simulink model "SCwith2SAsaug_ter"  (R2025b)
settings: Solver=VariableStepAuto  StartTime=0.0  StopTime=10.0  RelTol=1e-3
undefined symbols (not defined in the file): InvDyn, sig4, ureal, uss
libraries: RCTblocks x67
(part 1 of 2)
settings Model: Creator=d.alazard  LastModifiedBy=andre
settings SolverCC: AlgebraicLoopSolver=TrustRegion
settings DebuggingCC: AlgebraicLoopMsg=none  UnconnectedInputMsg=warning  UnconnectedOutputMsg=warning  UnconnectedLineMsg=warning
settings ModelReferenceCC: EnableRefExpFcnMdlSchedulingChecks=on
settings RTWCC: GPUComputeCapability=3.5  DLArmComputeVersion=19.05

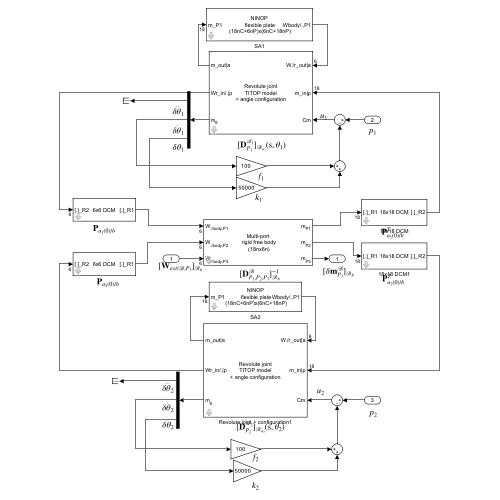
[thumbnail: Simulink's stored preview of the top-level diagram]
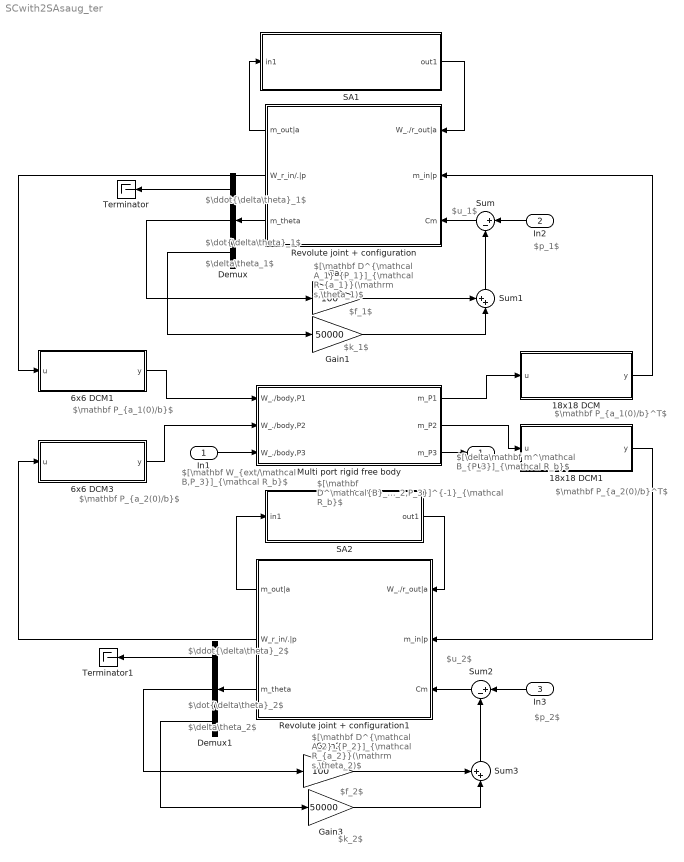
== system SCwith2SAsaug_ter ==
  note: $u_1$
  note: $\ddot{\delta\theta}_1$
  note: $\mathbf P_{a_1(0)/b}^T$
  note: $[\mathbf D^\mathcal{B}_{P_1,P_2,P_3}]^{-1}_{\mathcal R_b}$
  note: $\mathbf P_{a_1(0)/b}$
  note: $\mathbf P_{a_2(0)/b}$
  note: $\mathbf P_{a_2(0)/b}^T$
  note: $\dot{\delta\theta}_1$
  note: $\dot{\delta\theta}_2$
  note: $\ddot{\delta\theta}_2$
  note: $\delta\theta_1$
  note: $\delta\theta_2$
  note: $p_1$
  note: $u_2$
  note: $p_2$
  note: $f_1$
  note: $k_1$
  note: $k_2$
  note: $f_2$
  note: $[\mathbf D^{\mathcal A_1}_{P_1}]_{\mathcal R_{a_1}}(\mathrm s,\theta_1)$
  note: $[\mathbf D^{\mathcal A_2}_{P_2}]_{\mathcal R_{a_2}}(\mathrm s,\theta_2)$
  note: $[\mathbf W_{ext/\mathcal B,P_3}]_{\mathcal R_b}$
  note: $[\delta\mathbf m^\mathcal B_{P_3}]_{\mathcal R_b}$
  In1 : Inport
  In2 : Inport  Port=2
  In3 : Inport  Port=3
  18x18 DCM : Subsystem  mask(18x18 Direction cosine matrix (DCM)){rot=[0 -1 0;0 0 -1;1 0 0], transp=on}
      mask prompts: rot "3x3 DCM"; transp "Matrix transposed"
      mask help:
      | For 6 d.o.f. body motion vector (3 translations and 3 rotations, accelerations, velocities and positions), this block Implement the 18x18 rotation matrix (or its transposed) for a given 3x3 DCM.
      |
      | Considering 2 frames R1 and  R2, the DCM between R1 and R2 is defined as the 3x3 matrix where each column is the component vector of each R2 orthogonal unit vector expressed in R1. Thus
      |
      |    [v]_R1 = DCM  * [v]_R2.
      mask init:
      | if transp,
      |     rot=rot';
      | end
      mask Help: web('Doc18dcm.html','-browser')
      mask Display:
      | disp('18x18 DCM')
      | if transp
      |     port_label('input', 1, '[.]_R1')
      |     port_label('output', 1, '[.]_R2')
      | else
      |     port_label('input', 1, '[.]_R2')
      |     port_label('output', 1, '[.]_R1')
      | end
  18x18 DCM1 : Subsystem  mask(18x18 Direction cosine matrix (DCM)){rot=[0 1 0;0 0 -1;-1 0 0], transp=on}
      mask prompts: rot "3x3 DCM"; transp "Matrix transposed"
      mask help:
      | For 6 d.o.f. body motion vector (3 translations and 3 rotations, accelerations, velocities and positions), this block Implement the 18x18 rotation matrix (or its transposed) for a given 3x3 DCM.
      |
      | Considering 2 frames R1 and  R2, the DCM between R1 and R2 is defined as the 3x3 matrix where each column is the component vector of each R2 orthogonal unit vector expressed in R1. Thus
      |
      |    [v]_R1 = DCM  * [v]_R2.
      mask init:
      | if transp,
      |     rot=rot';
      | end
      mask Help: web('Doc18dcm.html','-browser')
      mask Display:
      | disp('18x18 DCM')
      | if transp
      |     port_label('input', 1, '[.]_R1')
      |     port_label('output', 1, '[.]_R2')
      | else
      |     port_label('input', 1, '[.]_R2')
      |     port_label('output', 1, '[.]_R1')
      | end
  6x6 DCM1 : Subsystem  mask(6x6 Direction cosine matrix (DCM)){rot=[0 -1 0;0 0 -1;1 0 0], transp=off}
      mask prompts: rot "3x3 DCM"; transp "Matrix transposed"
      mask help:
      | For 6 d.o.f. body motion (3 translations and 3 rotations), this block Implement the 6x6 rotation matrix (or its transposed) for a given 3x3 DCM.
      |
      | Considering 2 frames R1 and  R2, the DCM between R1 and R2 is defined as the 3x3 matrix where each column is the component vector of each R2 orthogonal unit vector expressed in R1. Thus
      |
      |    [v]_R1 = DCM  * [v]_R2.
      mask init:
      | if transp,
      |     rot=rot';
      | end
      mask Help: web('Doc6dcm.html','-browser')
      mask Display:
      | disp('6x6 DCM')
      | if transp
      |     port_label('input', 1, '[.]_R1')
      |     port_label('output', 1, '[.]_R2')
      | else
      |     port_label('input', 1, '[.]_R2')
      |     port_label('output', 1, '[.]_R1')
      | end
  6x6 DCM3 : Subsystem  mask(6x6 Direction cosine matrix (DCM)){rot=[0 1 0;0 0 -1;-1 0 0], transp=off}
      mask prompts: rot "3x3 DCM"; transp "Matrix transposed"
      mask help:
      | For 6 d.o.f. body motion (3 translations and 3 rotations), this block Implement the 6x6 rotation matrix (or its transposed) for a given 3x3 DCM.
      |
      | Considering 2 frames R1 and  R2, the DCM between R1 and R2 is defined as the 3x3 matrix where each column is the component vector of each R2 orthogonal unit vector expressed in R1. Thus
      |
      |    [v]_R1 = DCM  * [v]_R2.
      mask init:
      | if transp,
      |     rot=rot';
      | end
      mask Help: web('Doc6dcm.html','-browser')
      mask Display:
      | disp('6x6 DCM')
      | if transp
      |     port_label('input', 1, '[.]_R1')
      |     port_label('output', 1, '[.]_R2')
      | else
      |     port_label('input', 1, '[.]_R2')
      |     port_label('output', 1, '[.]_R1')
      | end
  Demux : Demux  Outputs=3
  Demux1 : Demux  Outputs=3
  Gain : Gain  Gain=100
  Gain1 : Gain  Gain=50000
  Gain2 : Gain  Gain=100
  Gain3 : Gain  Gain=50000
  Multi port rigid free body : Subsystem  mask(Multi-port rigid body (18nx6n)){m=1000, Ig=[75 1 2;1 40 -1;2 -1 80], OG=[0.35;1.5;0.5], n=3, OP1=[0.4;1.4;1], OP2=[0.4;1.4;0], OP3=[0.35;1.5;0.5], OP4=[0;0;0], OP5=[0;0;0]}
      mask prompts: m "Mass (Kg)"; Ig "Inertia (at G, Kg m^2)"; OG "OG (3x1 vector, m)"; n "Number of ports"; OP1 "OP1 (3x1 vector, m)"; OP2 "OP2 (3x1 vector, m)"; OP3 "OP3 (3x1 vector, m)"; OP4 "OP4 (3x1 vector, m)"; OP5 "OP5 (3x1 vector,m)"
      mask help:
      | 18nx6n dynamic model of a rigid body at n given points (ports) between wrenches applied at the n points (input) and the motions vectors at these points (output).
      |
      | 0: the reference point
      | G: the center of mass
      | Pi (i=1:n): the n given connection points (n<6).
      |
      | All parameters are expressed in the body frame.
      | Each parameter can be an uncertain parameter declared with "ureal"
      mask init:
      | MultiPortRigidFreeBody
      mask Help: web('Docmultiportrigidbase.html','-browser')
      mask TypeOptions n: 1 | 2 | 3 | 4 | 5
      mask DialogControl ParameterGroupVar Prompt: Main parameters
      mask DialogControl port1 Prompt: Port #1
      mask DialogControl port2 Prompt: #2
      mask DialogControl port3 Prompt: #3
      mask DialogControl port4 Prompt: #4
      mask DialogControl port5 Prompt: #5
      mask Display:
      | disp('Multi-port\n rigid free body\n (18nx6n)')
      | for ii=1:n
      |     port_label('input', ii,['W_{./body,P',num2str(ii),'}'],'interpreter','tex')
      |     port_label('output',ii,['m_{P',num2str(ii),'}'],'interpreter','tex')
      | end
  Revolute joint + configuration : Subsystem  mask(Revolute joint){ra=[1;0;0], Jr=1e-9, theta=ureal('Theta',0,'Range',[-pi pi])}
      mask prompts: ra "Direction of the joint in the local frame (3x1 vector)"; Jr "Rotor inertia (kg.m^2)"; theta "Angular configuration (rad)"
      mask help:
      | This block implement the TITOP model of of a revolute joint.
      | The last channel is the transfer between the torque applied inside the joint by the input shaft to the output shaft and the relative angular acceleration of the output shaft w.r.t the input shaft.
      |
      | Angular configuration can be a vayring parameter: Ex:
      | ureal('NAME',0,'Range',[-pi pi])
      |
      | Then, ULINEARIZE will provide a model involving the block named "tan_NAME_div4";
      mask init:
      | pass=ra2DCMi(ra);
      | ran=[ra(1);ra(2);ra(3)]/norm(ra);
      mask Help: web('DocRevoluteJoint_configuration.html','-browser')
      mask Display:
      | disp('Revolute joint\nTITOP model\n+ angle configuration')
      | port_label('input', 1, 'W./r_out|a')
      | port_label('output', 1, 'm_out|a')
      | port_label('input', 2, 'm_in|p')
      | port_label('output', 2, 'Wr_in/.|p')
      | port_label('input', 3, 'Cm')
      | port_label('output', 3, 'm_\theta','interpreter','tex')
  Revolute joint + configuration1 : Subsystem  mask(Revolute joint){ra=[-1;0;0], Jr=1e-9, theta=ureal('Theta',0,'Range',[-pi pi])}
      mask prompts: ra "Direction of the joint in the local frame (3x1 vector)"; Jr "Rotor inertia (kg.m^2)"; theta "Angular configuration (rad)"
      mask help:
      | This block implement the TITOP model of of a revolute joint.
      | The last channel is the transfer between the torque applied inside the joint by the input shaft to the output shaft and the relative angular acceleration of the output shaft w.r.t the input shaft.
      |
      | Angular configuration can be a vayring parameter: Ex:
      | ureal('NAME',0,'Range',[-pi pi])
      |
      | Then, ULINEARIZE will provide a model involving the block named "tan_NAME_div4";
      mask init:
      | pass=ra2DCMi(ra);
      | ran=[ra(1);ra(2);ra(3)]/norm(ra);
      mask Help: web('DocRevoluteJoint_configuration.html','-browser')
      mask Display:
      | disp('Revolute joint\nTITOP model\n+ angle configuration')
      | port_label('input', 1, 'W./r_out|a')
      | port_label('output', 1, 'm_out|a')
      | port_label('input', 2, 'm_in|p')
      | port_label('output', 2, 'Wr_in/.|p')
      | port_label('input', 3, 'Cm')
      | port_label('output', 3, 'm_\theta','interpreter','tex')
  SA1 : Subsystem  mask(Multi-port flexible plate (18nC+6nP)x(6nC+18nP)){lx=4.14, ly=2.2, t=0.01, rho=474, E=44e9, ni=0.35, xi=0.005, i_nP=1, i_nC=0, OP1=[0;1.1;0], OP2=[4.14;1.1;0], OP3=[4.14;0;0], OP4=[4.14;2.2;0], OC1=[4.14;2.2;0], OC2=[0;0;0], OC3=[4.14;0;0], OC4=[4.14;2.2;0], OC5=[4.14;1.1;0], OC6=[0;1.1;0], OC7=[0;0;0], OC8=[0;0;0], RedSlowOn=off, uw_var=5, Nflex=0}
      mask prompts: lx "lenght along x (m)"; ly "length along y (m)"; t "thickness (m)"; rho "Mass density (Kg/m^3)"; E "Young modulus (N/m^2)"; ni "Poisson coefficient"; xi "damping coefficient"; i_nP "Number of parent (P) nodes (<5)"; i_nC "Number of child (C) nodes"; OP1 "OP1 (3x1 vector: [x;y;0], m)"; OP2 "OP2 (3x1 vectorr: [x;y;0], m)"; OP3 "OP3 (3x1 vectorr: [x;y;0], m)"; OP4 "OP4 (3x1 vectorr: [x;y;0], m)"; OC1 "OC1 (3x1 vectorr: [x;y;0], m)"; OC2 "OC2 (3x1 vectorr: [x;y;0], m)"; OC3 "OC3 (3x1 vectorr: [x;y;0], m)"; OC4 "OC4 (3x1 vectorr: [x;y;0], m)"; OC5 "OC5 (3x1 vectorr: [x;y;0], m)"; OC6 "OC6 (3x1 vectorr: [x;y;0], m)"; OC7 "OC7 (3x1 vector: [x;y;0],m)"; OC8 "OC8 (3x1 vector [x;y;0], m)"; RedSlowOn "Reduction of the 6*(nP-1) poles at 0 (due to loop closure constraints when nP>1)."; uw_var "uncertainty (%)"; Nflex "number of flexible modes (Nf, integer)"
      mask help:
      | (18nC+6nP)x(6nC+18nP) multi-port model of a uniform plate (in the x-y plane) between
      |   *  wrenches applied to the plate at the given nC child nodes (input) and motion vectors at these child nodes (output)
      |   *  motion vectors at the nP parent nodes (input)  and wrenches applied by this plate at these parent nodes (output)
      |  dynamic model of a uniform flexible plate (in the x-y plane),
      | in the plate reference frame (0,x,y,z)
      |
      | The plate is defined by:
      | * 0<x<lx
      | * 0<y<ly
      | * -t/2<z<t/2
      |
      | All parameters are expressed in the plate reference frame.
      | Dynamics in translations along x and y and rotation around z are assumed rigid.
      mask init:
      | MultiPortFlexiblePlateAug
      mask Help: web('DocPlate_joly.html','-browser')
      mask TypeOptions i_nP: 0 | 1 | 2 | 3 | 4
      mask TypeOptions i_nC: 0 | 1 | 2 | 3 | 4 | 5 | 6 | 7 | 8
      mask DialogControl ParameterGroupVar Prompt: Main parameters
      mask DialogControl Pport1 Prompt: P node #1
      mask DialogControl Pport2 Prompt: #2
      mask DialogControl Pport3 Prompt: #3
      mask DialogControl Pport4 Prompt: #4
      mask DialogControl Cport1 Prompt: C node #1
      mask DialogControl Cport2 Prompt: #2
      mask DialogControl Cport3 Prompt: #3
      mask DialogControl Cport4 Prompt: #4
      mask DialogControl Cport5 Prompt: #5
      mask DialogControl Cport6 Prompt: #6
      mask DialogControl Cport7 Prompt: #7
      mask DialogControl Cport8 Prompt: #8
      mask DialogControl Reduction Prompt: Optional Reduction
      mask DialogControl Container19 Prompt: Parametric uncertainties
      mask DialogControl Control8 Prompt: The uncertain parameters are the first Nf cantilevered frequencies of the plate when it is clamped at the first parent node (P1) or the last child node when the number of parent nodes is null.
      mask DialogControl Control4 Prompt: The uncertain frequency is named: 'w_name_i' where:
      mask DialogControl Control5 Prompt: * 'name' is the current block name (reduced to its alphanumeric characters).
      mask DialogControl Control6 Prompt: * 'i' is the flexible mode number (increasing frequency order)
      mask Display:
      | disp('NINOP\n flexible plate\n (18nC+6nP)x(6nC+18nP)')
      | if nC~=0
      |     for ii=1:nC
      |         port_label('input', ii, ['W./body,C',num2str(ii)])
      |         port_label('output',ii,['m_C',num2str(ii)])
      |     end
      | end
      | if nP~=0
      |     for ii=1:nP
      |         port_label('input', nC+ii, ['m_P',num2str(ii)])
      |         port_label('output',nC+ii,['Wbody/.,P',num2str(ii)])
      |     end
      | end
  SA2 : Subsystem  mask(Multi-port flexible plate (18nC+6nP)x(6nC+18nP)){lx=4.14, ly=2.2, t=0.01, rho=474, E=44e9, ni=0.35, xi=0.005, i_nP=1, i_nC=0, OP1=[0;1.1;0], OP2=[4.14;1.1;0], OP3=[4.14;0;0], OP4=[4.14;2.2;0], OC1=[4.14;2.2;0], OC2=[0;0;0], OC3=[4.14;0;0], OC4=[4.14;2.2;0], OC5=[4.14;1.1;0], OC6=[0;1.1;0], OC7=[0;0;0], OC8=[0;0;0], RedSlowOn=off, uw_var=5, Nflex=0}
      mask prompts: lx "lenght along x (m)"; ly "length along y (m)"; t "thickness (m)"; rho "Mass density (Kg/m^3)"; E "Young modulus (N/m^2)"; ni "Poisson coefficient"; xi "damping coefficient"; i_nP "Number of parent (P) nodes (<5)"; i_nC "Number of child (C) nodes"; OP1 "OP1 (3x1 vector: [x;y;0], m)"; OP2 "OP2 (3x1 vectorr: [x;y;0], m)"; OP3 "OP3 (3x1 vectorr: [x;y;0], m)"; OP4 "OP4 (3x1 vectorr: [x;y;0], m)"; OC1 "OC1 (3x1 vectorr: [x;y;0], m)"; OC2 "OC2 (3x1 vectorr: [x;y;0], m)"; OC3 "OC3 (3x1 vectorr: [x;y;0], m)"; OC4 "OC4 (3x1 vectorr: [x;y;0], m)"; OC5 "OC5 (3x1 vectorr: [x;y;0], m)"; OC6 "OC6 (3x1 vectorr: [x;y;0], m)"; OC7 "OC7 (3x1 vector: [x;y;0],m)"; OC8 "OC8 (3x1 vector [x;y;0], m)"; RedSlowOn "Reduction of the 6*(nP-1) poles at 0 (due to loop closure constraints when nP>1)."; uw_var "uncertainty (%)"; Nflex "number of flexible modes (Nf, integer)"
      mask help:
      | (18nC+6nP)x(6nC+18nP) multi-port model of a uniform plate (in the x-y plane) between
      |   *  wrenches applied to the plate at the given nC child nodes (input) and motion vectors at these child nodes (output)
      |   *  motion vectors at the nP parent nodes (input)  and wrenches applied by this plate at these parent nodes (output)
      |  dynamic model of a uniform flexible plate (in the x-y plane),
      | in the plate reference frame (0,x,y,z)
      |
      | The plate is defined by:
      | * 0<x<lx
      | * 0<y<ly
      | * -t/2<z<t/2
      |
      | All parameters are expressed in the plate reference frame.
      | Dynamics in translations along x and y and rotation around z are assumed rigid.
      mask init:
      | MultiPortFlexiblePlateAug
      mask Help: web('DocPlate_joly.html','-browser')
      mask TypeOptions i_nP: 0 | 1 | 2 | 3 | 4
      mask TypeOptions i_nC: 0 | 1 | 2 | 3 | 4 | 5 | 6 | 7 | 8
      mask DialogControl ParameterGroupVar Prompt: Main parameters
      mask DialogControl Pport1 Prompt: P node #1
      mask DialogControl Pport2 Prompt: #2
      mask DialogControl Pport3 Prompt: #3
      mask DialogControl Pport4 Prompt: #4
      mask DialogControl Cport1 Prompt: C node #1
      mask DialogControl Cport2 Prompt: #2
      mask DialogControl Cport3 Prompt: #3
      mask DialogControl Cport4 Prompt: #4
      mask DialogControl Cport5 Prompt: #5
      mask DialogControl Cport6 Prompt: #6
      mask DialogControl Cport7 Prompt: #7
      mask DialogControl Cport8 Prompt: #8
      mask DialogControl Reduction Prompt: Optional Reduction
      mask DialogControl Container19 Prompt: Parametric uncertainties
      mask DialogControl Control8 Prompt: The uncertain parameters are the first Nf cantilevered frequencies of the plate when it is clamped at the first parent node (P1) or the last child node when the number of parent nodes is null.
      mask DialogControl Control4 Prompt: The uncertain frequency is named: 'w_name_i' where:
      mask DialogControl Control5 Prompt: * 'name' is the current block name (reduced to its alphanumeric characters).
      mask DialogControl Control6 Prompt: * 'i' is the flexible mode number (increasing frequency order)
      mask Display:
      | disp('NINOP\n flexible plate\n (18nC+6nP)x(6nC+18nP)')
      | if nC~=0
      |     for ii=1:nC
      |         port_label('input', ii, ['W./body,C',num2str(ii)])
      |         port_label('output',ii,['m_C',num2str(ii)])
      |     end
      | end
      | if nP~=0
      |     for ii=1:nP
      |         port_label('input', nC+ii, ['m_P',num2str(ii)])
      |         port_label('output',nC+ii,['Wbody/.,P',num2str(ii)])
      |     end
      | end
  Sum : Sum  Inputs=|+-
  Sum1 : Sum  Inputs=++|
  Sum2 : Sum  Inputs=|+-
  Sum3 : Sum  Inputs=++|
  Terminator : Terminator
  Terminator1 : Terminator
  Out1 : Outport
  wires:
  6x6 DCM1/1(y) -> Multi port rigid free body/1(W_./body,P1)
  Multi port rigid free body/1(m_P1) -> 18x18 DCM/1(u)
  6x6 DCM3/1(y) -> Multi port rigid free body/2(W_./body,P2)
  Multi port rigid free body/2(m_P2) -> 18x18 DCM1/1(u)
  18x18 DCM/1(y) -> Revolute joint + configuration/2(m_in|p)
  Revolute joint + configuration/2(W_r_in/.|p) -> 6x6 DCM1/1(u)
  18x18 DCM1/1(y) -> Revolute joint + configuration1/2(m_in|p)
  Revolute joint + configuration1/2(W_r_in/.|p) -> 6x6 DCM3/1(u)
  In1/1 -> Multi port rigid free body/3(W_./body,P3)
  Multi port rigid free body/3(m_P3) -> Out1/1
  Demux/3 -> Gain1/1
  In2/1 -> Sum/1
  Gain/1 -> Sum1/1
  Gain1/1 -> Sum1/2
  Sum1/1 -> Sum/2
  Sum/1 -> Revolute joint + configuration/3(Cm)
  Gain2/1 -> Sum3/1
  Sum3/1 -> Sum2/2
  In3/1 -> Sum2/1
  Sum2/1 -> Revolute joint + configuration1/3(Cm)
  Gain3/1 -> Sum3/2
  Revolute joint + configuration/3(m_theta) -> Demux/1
  Demux/2 -> Gain/1
  Demux/1 -> Terminator/1
  Demux1/1 -> Terminator1/1
  Revolute joint + configuration1/3(m_theta) -> Demux1/1
  Demux1/3 -> Gain3/1
  Demux1/2 -> Gain2/1
  SA2/1(out1) -> Revolute joint + configuration1/1(W_./r_out|a)
  Revolute joint + configuration1/1(m_out|a) -> SA2/1(in1)
  SA1/1(out1) -> Revolute joint + configuration/1(W_./r_out|a)
  Revolute joint + configuration/1(m_out|a) -> SA1/1(in1)

== system SCwith2SAsaug_ter/18x18 DCM ==
  u : Inport  PortDimensions=18
  Demux : Demux  Outputs=[3 3 3 3 3 3]
  Mux : Mux  Inputs=[3 3 3 3 3 3]
  rotation : Gain  Gain=rot  Multiplication=Matrix(K*u) (u vector)
  rotation1 : Gain  Gain=rot  Multiplication=Matrix(K*u) (u vector)
  rotation2 : Gain  Gain=rot  Multiplication=Matrix(K*u) (u vector)
  translation : Gain  Gain=rot  Multiplication=Matrix(K*u) (u vector)
  translation1 : Gain  Gain=rot  Multiplication=Matrix(K*u) (u vector)
  translation2 : Gain  Gain=rot  Multiplication=Matrix(K*u) (u vector)
  y : Outport  VectorParamsAs1DForOutWhenUnconnected=off
  wires:
  Demux/6 -> rotation2/1
  rotation2/1 -> Mux/6
  translation2/1 -> Mux/5
  Demux/5 -> translation2/1
  rotation1/1 -> Mux/4
  translation1/1 -> Mux/3
  Demux/3 -> translation1/1
  Demux/4 -> rotation1/1
  Demux/2 -> rotation/1
  Mux/1 -> y/1
  u/1 -> Demux/1
  Demux/1 -> translation/1
  translation/1 -> Mux/1
  rotation/1 -> Mux/2

== system SCwith2SAsaug_ter/18x18 DCM1 ==
  u : Inport  PortDimensions=18
  Demux : Demux  Outputs=[3 3 3 3 3 3]
  Mux : Mux  Inputs=[3 3 3 3 3 3]
  rotation : Gain  Gain=rot  Multiplication=Matrix(K*u) (u vector)
  rotation1 : Gain  Gain=rot  Multiplication=Matrix(K*u) (u vector)
  rotation2 : Gain  Gain=rot  Multiplication=Matrix(K*u) (u vector)
  translation : Gain  Gain=rot  Multiplication=Matrix(K*u) (u vector)
  translation1 : Gain  Gain=rot  Multiplication=Matrix(K*u) (u vector)
  translation2 : Gain  Gain=rot  Multiplication=Matrix(K*u) (u vector)
  y : Outport  VectorParamsAs1DForOutWhenUnconnected=off
  wires:
  Demux/6 -> rotation2/1
  rotation2/1 -> Mux/6
  translation2/1 -> Mux/5
  Demux/5 -> translation2/1
  rotation1/1 -> Mux/4
  translation1/1 -> Mux/3
  Demux/3 -> translation1/1
  Demux/4 -> rotation1/1
  Demux/2 -> rotation/1
  Mux/1 -> y/1
  u/1 -> Demux/1
  Demux/1 -> translation/1
  translation/1 -> Mux/1
  rotation/1 -> Mux/2

== system SCwith2SAsaug_ter/6x6 DCM1 ==
  u : Inport  PortDimensions=6
  Demux : Demux  Outputs=[3 3]
  Mux : Mux  Inputs=[3 3]
  rotation : Gain  Gain=rot  Multiplication=Matrix(K*u) (u vector)
  translation : Gain  Gain=rot  Multiplication=Matrix(K*u) (u vector)
  y : Outport  VectorParamsAs1DForOutWhenUnconnected=off
  wires:
  rotation/1 -> Mux/2
  translation/1 -> Mux/1
  Demux/1 -> translation/1
  u/1 -> Demux/1
  Mux/1 -> y/1
  Demux/2 -> rotation/1

== system SCwith2SAsaug_ter/6x6 DCM3 ==
  u : Inport  PortDimensions=6
  Demux : Demux  Outputs=[3 3]
  Mux : Mux  Inputs=[3 3]
  rotation : Gain  Gain=rot  Multiplication=Matrix(K*u) (u vector)
  translation : Gain  Gain=rot  Multiplication=Matrix(K*u) (u vector)
  y : Outport  VectorParamsAs1DForOutWhenUnconnected=off
  wires:
  rotation/1 -> Mux/2
  translation/1 -> Mux/1
  Demux/1 -> translation/1
  u/1 -> Demux/1
  Mux/1 -> y/1
  Demux/2 -> rotation/1

== system SCwith2SAsaug_ter/Multi port rigid free body ==
  W_./body,P1 : Inport  PortDimensions=6
  W_./body,P2 : Inport  Port=2  PortDimensions=6
  W_./body,P3 : Inport  Port=3  PortDimensions=6
  Demux : Demux  Outputs=[18 18 18]
      settings: DisplayOption=none
  Gain : RCTblocks/Uncertain State Space  Tag=USS  USystem=uss(InvDyn)  UValue=[]  X0=[]  uX0=[]
  Mux : Mux  Inputs=[6 6 6]
  m_P1 : Outport
  m_P2 : Outport  Port=2
  m_P3 : Outport  Port=3
  wires:
  Demux/3 -> m_P3/1
  W_./body,P3/1 -> Mux/3
  Demux/2 -> m_P2/1
  W_./body,P2/1 -> Mux/2
  Demux/1 -> m_P1/1
  W_./body,P1/1 -> Mux/1
  Gain/1 -> Demux/1
  Mux/1 -> Gain/1

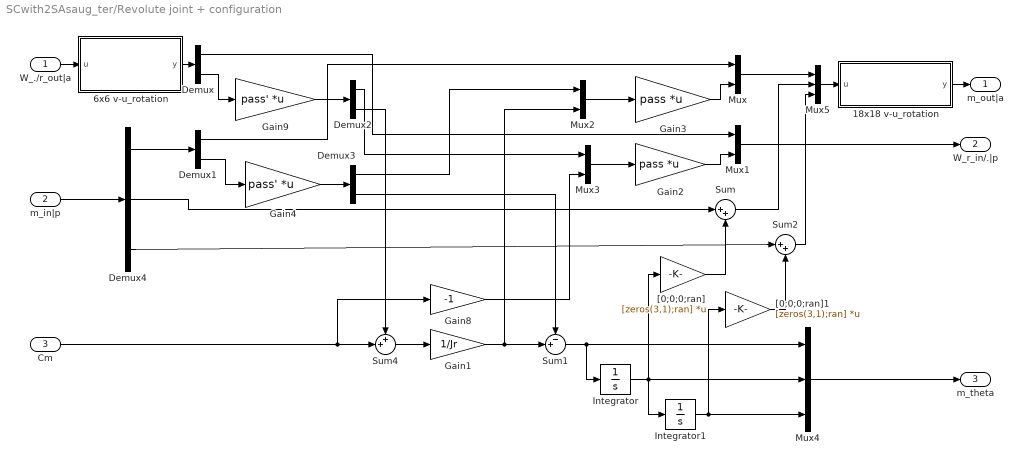
== system SCwith2SAsaug_ter/Revolute joint + configuration ==
  W_./r_out|a : Inport  PortDimensions=6
  m_in|p : Inport  Port=2  PortDimensions=18
  Cm : Inport  Port=3  PortDimensions=1
  18x18 v-u_rotation : Subsystem  mask(18x18 rotation matrix (around a given axis)){ra=ra, theta=theta, transp=on}
      mask prompts: ra "Rotation axis (3x1 vector)"; theta "Angle (rad)"; transp "Matrix transposed"
      mask help:
      | For 6 d.o.f. body motion vector (3 translations and 3 rotations, acceleration velocities and positions), this block Implement the 18x18 rotation matrix (or its transposed)  for a given angle around a given axis.
      |
      | Angle  (rad) can be an uncertain parameter declared with "ureal" with mode 'Range'
      | Ex: ureal('NAME',0,'Range',[-pi pi])
      | Then, ULINEARIZE will provide a model involving the block named "tan_NAME_div4".
      mask init:
      | vUrotation3x3
      mask Help: web('Doc6vurotation.html','-browser')
      mask Display:
      | disp('v-rot\n18x18')
      | if transp
      |     port_label('input', 1, '[.]_R1')
      |     port_label('output', 1, '[.]_R2')
      | else
      |     port_label('input', 1, '[.]_R2')
      |     port_label('output', 1, '[.]_R1')
      | end
  6x6 v-u_rotation : Subsystem  mask(6x6 rotation matrix (around a given axis)){ra=ra, theta=theta, transp=off}
      mask prompts: ra "Rotation axis (3x1 vector)"; theta "Angle (rad)"; transp "Matrix transposed"
      mask help:
      | For 6 d.o.f. body motion (3 translations and 3 rotations), this block Implement the 6x6 rotation matrix (or its transposed) for a given angle around a given axis.
      |
      | Angle  (rad) can be an uncertain parameter declared with "ureal" with mode 'Range'
      | Ex: ureal('NAME',0,'Range',[-pi pi])
      | Then, ULINEARIZE will provide a model involving the block named "tan_NAME_div4".
      mask init:
      | vUrotation3x3
      mask Help: web('Doc6vurotation.html','-browser')
      mask Display:
      | disp('v-rot\n6x6')
      | if transp
      |     port_label('input', 1, '[.]_R1')
      |     port_label('output', 1, '[.]_R2')
      | else
      |     port_label('input', 1, '[.]_R2')
      |     port_label('output', 1, '[.]_R1')
      | end
  Demux : Demux  Outputs=[3 3]
  Demux1 : Demux  Outputs=[3 3]
  Demux2 : Demux  Outputs=[2 1]
  Demux3 : Demux  Outputs=[2 1]
  Demux4 : Demux  Outputs=[6 6 6]
  Gain1 : Gain  Gain=1/Jr
  Gain2 : Gain  Gain=pass  Multiplication=Matrix(K*u) (u vector)
  Gain3 : Gain  Gain=pass  Multiplication=Matrix(K*u) (u vector)
  Gain4 : Gain  Gain=pass'  Multiplication=Matrix(K*u) (u vector)
  Gain8 : Gain  Gain=-1
  Gain9 : Gain  Gain=pass'  Multiplication=Matrix(K*u) (u vector)
  Integrator : Integrator
  Integrator1 : Integrator
  Mux : Mux  Inputs=[3 3]
  Mux1 : Mux  Inputs=[3 3]
  Mux2 : Mux  Inputs=[2 1]
  Mux3 : Mux  Inputs=[2 1]
  Mux4 : Mux  Inputs=3
  Mux5 : Mux  Inputs=[6 6 6]
  Sum : Sum  Inputs=|++
  Sum1 : Sum  Inputs=-+|
  Sum2 : Sum  Inputs=|++
  Sum4 : Sum  Inputs=++|
  "[0;0;0;ran]" : Gain  Gain=[zeros(3,1);ran]  Multiplication=Matrix(K*u) (u vector)
  "[0;0;0;ran]1" : Gain  Gain=[zeros(3,1);ran]  Multiplication=Matrix(K*u) (u vector)
  m_out|a : Outport  VectorParamsAs1DForOutWhenUnconnected=off
  W_r_in/.|p : Outport  Port=2  VectorParamsAs1DForOutWhenUnconnected=off
  m_theta : Outport  Port=3  VectorParamsAs1DForOutWhenUnconnected=off
  wires:
  Sum2/1 -> Mux5/3
  Sum/1 -> Mux5/2
  Mux5/1 -> 18x18 v-u_rotation/1(u)
  Mux/1 -> Mux5/1
  Demux4/3 -> Sum2/1
  Demux4/2 -> Sum/1
  "[0;0;0;ran]1"/1 -> Sum2/2
  "[0;0;0;ran]"/1 -> Sum/2
  Integrator1/1 -> Mux4/3, "[0;0;0;ran]1"/1
  Sum1/1 -> Mux4/1, Integrator/1
  Mux4/1 -> m_theta/1
  Integrator/1 -> Integrator1/1, Mux4/2, "[0;0;0;ran]"/1
  m_in|p/1 -> Demux4/1
  Demux4/1 -> Demux1/1
  W_./r_out|a/1 -> 6x6 v-u_rotation/1(u)
  Mux1/1 -> W_r_in/.|p/1
  Demux1/1 -> Mux/1
  Cm/1 -> Gain8/1, Sum4/2
  Demux/1 -> Mux1/1
  Gain2/1 -> Mux1/2
  Demux/2 -> Gain9/1
  Gain1/1 -> Mux2/2, Sum1/2
  Sum4/1 -> Gain1/1
  Gain3/1 -> Mux/2
  Demux3/2 -> Sum1/1
  Gain9/1 -> Demux2/1
  Demux2/2 -> Sum4/1
  Mux2/1 -> Gain3/1
  Demux1/2 -> Gain4/1
  Gain4/1 -> Demux3/1
  Mux3/1 -> Gain2/1
  Gain8/1 -> Mux3/2
  Demux2/1 -> Mux3/1
  Demux3/1 -> Mux2/1
  6x6 v-u_rotation/1(y) -> Demux/1
  18x18 v-u_rotation/1(y) -> m_out|a/1

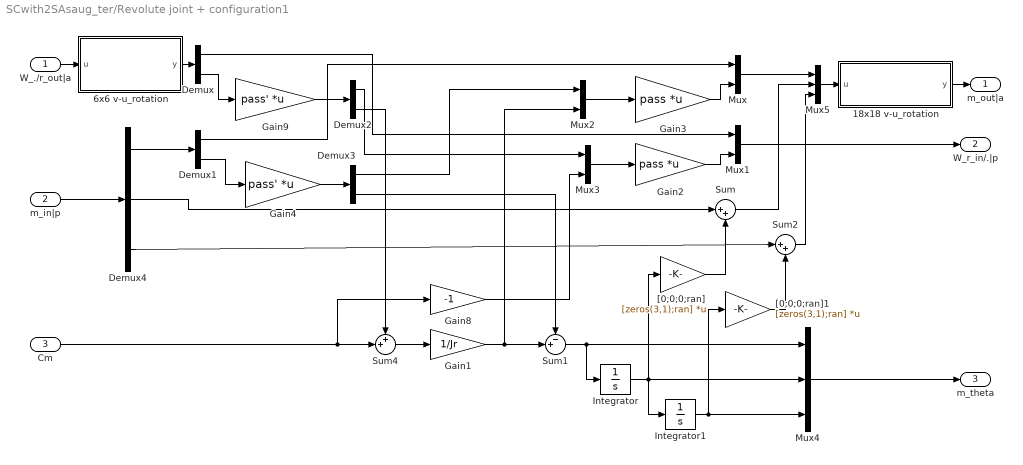
== system SCwith2SAsaug_ter/Revolute joint + configuration1 ==
  W_./r_out|a : Inport  PortDimensions=6
  m_in|p : Inport  Port=2  PortDimensions=18
  Cm : Inport  Port=3  PortDimensions=1
  18x18 v-u_rotation : Subsystem  mask(18x18 rotation matrix (around a given axis)){ra=ra, theta=theta, transp=on}
      mask prompts: ra "Rotation axis (3x1 vector)"; theta "Angle (rad)"; transp "Matrix transposed"
      mask help:
      | For 6 d.o.f. body motion vector (3 translations and 3 rotations, acceleration velocities and positions), this block Implement the 18x18 rotation matrix (or its transposed)  for a given angle around a given axis.
      |
      | Angle  (rad) can be an uncertain parameter declared with "ureal" with mode 'Range'
      | Ex: ureal('NAME',0,'Range',[-pi pi])
      | Then, ULINEARIZE will provide a model involving the block named "tan_NAME_div4".
      mask init:
      | vUrotation3x3
      mask Help: web('Doc6vurotation.html','-browser')
      mask Display:
      | disp('v-rot\n18x18')
      | if transp
      |     port_label('input', 1, '[.]_R1')
      |     port_label('output', 1, '[.]_R2')
      | else
      |     port_label('input', 1, '[.]_R2')
      |     port_label('output', 1, '[.]_R1')
      | end
  6x6 v-u_rotation : Subsystem  mask(6x6 rotation matrix (around a given axis)){ra=ra, theta=theta, transp=off}
      mask prompts: ra "Rotation axis (3x1 vector)"; theta "Angle (rad)"; transp "Matrix transposed"
      mask help:
      | For 6 d.o.f. body motion (3 translations and 3 rotations), this block Implement the 6x6 rotation matrix (or its transposed) for a given angle around a given axis.
      |
      | Angle  (rad) can be an uncertain parameter declared with "ureal" with mode 'Range'
      | Ex: ureal('NAME',0,'Range',[-pi pi])
      | Then, ULINEARIZE will provide a model involving the block named "tan_NAME_div4".
      mask init:
      | vUrotation3x3
      mask Help: web('Doc6vurotation.html','-browser')
      mask Display:
      | disp('v-rot\n6x6')
      | if transp
      |     port_label('input', 1, '[.]_R1')
      |     port_label('output', 1, '[.]_R2')
      | else
      |     port_label('input', 1, '[.]_R2')
      |     port_label('output', 1, '[.]_R1')
      | end
  Demux : Demux  Outputs=[3 3]
  Demux1 : Demux  Outputs=[3 3]
  Demux2 : Demux  Outputs=[2 1]
  Demux3 : Demux  Outputs=[2 1]
  Demux4 : Demux  Outputs=[6 6 6]
  Gain1 : Gain  Gain=1/Jr
  Gain2 : Gain  Gain=pass  Multiplication=Matrix(K*u) (u vector)
  Gain3 : Gain  Gain=pass  Multiplication=Matrix(K*u) (u vector)
  Gain4 : Gain  Gain=pass'  Multiplication=Matrix(K*u) (u vector)
  Gain8 : Gain  Gain=-1
  Gain9 : Gain  Gain=pass'  Multiplication=Matrix(K*u) (u vector)
  Integrator : Integrator
  Integrator1 : Integrator
  Mux : Mux  Inputs=[3 3]
  Mux1 : Mux  Inputs=[3 3]
  Mux2 : Mux  Inputs=[2 1]
  Mux3 : Mux  Inputs=[2 1]
  Mux4 : Mux  Inputs=3
  Mux5 : Mux  Inputs=[6 6 6]
  Sum : Sum  Inputs=|++
  Sum1 : Sum  Inputs=-+|
  Sum2 : Sum  Inputs=|++
  Sum4 : Sum  Inputs=++|
  "[0;0;0;ran]" : Gain  Gain=[zeros(3,1);ran]  Multiplication=Matrix(K*u) (u vector)
  "[0;0;0;ran]1" : Gain  Gain=[zeros(3,1);ran]  Multiplication=Matrix(K*u) (u vector)
  m_out|a : Outport  VectorParamsAs1DForOutWhenUnconnected=off
  W_r_in/.|p : Outport  Port=2  VectorParamsAs1DForOutWhenUnconnected=off
  m_theta : Outport  Port=3  VectorParamsAs1DForOutWhenUnconnected=off
  wires:
  18x18 v-u_rotation/1(y) -> m_out|a/1
  6x6 v-u_rotation/1(y) -> Demux/1
  Demux3/1 -> Mux2/1
  Demux2/1 -> Mux3/1
  Gain8/1 -> Mux3/2
  Mux3/1 -> Gain2/1
  Gain4/1 -> Demux3/1
  Demux1/2 -> Gain4/1
  Mux2/1 -> Gain3/1
  Demux2/2 -> Sum4/1
  Gain9/1 -> Demux2/1
  Demux3/2 -> Sum1/1
  Gain3/1 -> Mux/2
  Sum4/1 -> Gain1/1
  Gain1/1 -> Sum1/2, Mux2/2
  Demux/2 -> Gain9/1
  Gain2/1 -> Mux1/2
  Demux/1 -> Mux1/1
  Cm/1 -> Sum4/2, Gain8/1
  Demux1/1 -> Mux/1
  Mux1/1 -> W_r_in/.|p/1
  W_./r_out|a/1 -> 6x6 v-u_rotation/1(u)
  Demux4/1 -> Demux1/1
  m_in|p/1 -> Demux4/1
  Integrator/1 -> "[0;0;0;ran]"/1, Mux4/2, Integrator1/1
  Mux4/1 -> m_theta/1
  Sum1/1 -> Integrator/1, Mux4/1
  Integrator1/1 -> "[0;0;0;ran]1"/1, Mux4/3
  "[0;0;0;ran]"/1 -> Sum/2
  "[0;0;0;ran]1"/1 -> Sum2/2
  Demux4/2 -> Sum/1
  Demux4/3 -> Sum2/1
  Mux/1 -> Mux5/1
  Mux5/1 -> 18x18 v-u_rotation/1(u)
  Sum/1 -> Mux5/2
  Sum2/1 -> Mux5/3

== system SCwith2SAsaug_ter/SA1 ==
  in1 : Inport  PortDimensions=18
  Demux : Demux  Outputs=[6 ]
  Mux : Mux  Inputs=[18 ]
  ninop : RCTblocks/Uncertain State Space  Tag=USS  USystem=NINOP  UValue=[]  X0=[]  uX0=[]
  out1 : Outport
  wires:
  Mux/1 -> ninop/1
  ninop/1 -> Demux/1
  in1/1 -> Mux/1
  Demux/1 -> out1/1

== system SCwith2SAsaug_ter/SA2 ==
  in1 : Inport  PortDimensions=18
  Demux : Demux  Outputs=[6 ]
  Mux : Mux  Inputs=[18 ]
  ninop : RCTblocks/Uncertain State Space  Tag=USS  USystem=NINOP  UValue=[]  X0=[]  uX0=[]
  out1 : Outport
  wires:
  Demux/1 -> out1/1
  in1/1 -> Mux/1
  ninop/1 -> Demux/1
  Mux/1 -> ninop/1

== system SCwith2SAsaug_ter/Revolute joint + configuration/18x18 v-u_rotation ==
  u : Inport  PortDimensions=18
  Demux : Demux  Outputs=[3 3 3 3 3 3]
  Mux : Mux  Inputs=[3 3 3 3 3 3]
  Subsystem : Subsystem
  Subsystem1 : Subsystem
  Subsystem2 : Subsystem
  Subsystem3 : Subsystem
  Subsystem4 : Subsystem
  Subsystem5 : Subsystem
  y : Outport  VectorParamsAs1DForOutWhenUnconnected=off
  wires:
  Subsystem5/1(Out1) -> Mux/6
  Demux/6 -> Subsystem5/1(In1)
  Subsystem4/1(Out1) -> Mux/5
  Demux/5 -> Subsystem4/1(In1)
  Subsystem3/1(Out1) -> Mux/4
  Demux/4 -> Subsystem3/1(In1)
  Subsystem2/1(Out1) -> Mux/3
  Demux/3 -> Subsystem2/1(In1)
  Mux/1 -> y/1
  u/1 -> Demux/1
  Demux/1 -> Subsystem/1(In1)
  Demux/2 -> Subsystem1/1(In1)
  Subsystem/1(Out1) -> Mux/1
  Subsystem1/1(Out1) -> Mux/2

== system SCwith2SAsaug_ter/Revolute joint + configuration/6x6 v-u_rotation ==
  u : Inport  PortDimensions=6
  Demux : Demux  Outputs=[3 3]
  Mux : Mux  Inputs=[3 3]
  Subsystem : Subsystem
  Subsystem1 : Subsystem
  y : Outport  VectorParamsAs1DForOutWhenUnconnected=off
  wires:
  Subsystem1/1(Out1) -> Mux/2
  Subsystem/1(Out1) -> Mux/1
  Demux/2 -> Subsystem1/1(In1)
  Demux/1 -> Subsystem/1(In1)
  u/1 -> Demux/1
  Mux/1 -> y/1

== system SCwith2SAsaug_ter/Revolute joint + configuration1/18x18 v-u_rotation ==
  u : Inport  PortDimensions=18
  Demux : Demux  Outputs=[3 3 3 3 3 3]
  Mux : Mux  Inputs=[3 3 3 3 3 3]
  Subsystem : Subsystem
  Subsystem1 : Subsystem
  Subsystem2 : Subsystem
  Subsystem3 : Subsystem
  Subsystem4 : Subsystem
  Subsystem5 : Subsystem
  y : Outport  VectorParamsAs1DForOutWhenUnconnected=off
  wires:
  Subsystem1/1(Out1) -> Mux/2
  Subsystem/1(Out1) -> Mux/1
  Demux/2 -> Subsystem1/1(In1)
  Demux/1 -> Subsystem/1(In1)
  u/1 -> Demux/1
  Mux/1 -> y/1
  Demux/3 -> Subsystem2/1(In1)
  Subsystem2/1(Out1) -> Mux/3
  Demux/4 -> Subsystem3/1(In1)
  Subsystem3/1(Out1) -> Mux/4
  Demux/5 -> Subsystem4/1(In1)
  Subsystem4/1(Out1) -> Mux/5
  Demux/6 -> Subsystem5/1(In1)
  Subsystem5/1(Out1) -> Mux/6

== system SCwith2SAsaug_ter/Revolute joint + configuration1/6x6 v-u_rotation ==
  u : Inport  PortDimensions=6
  Demux : Demux  Outputs=[3 3]
  Mux : Mux  Inputs=[3 3]
  Subsystem : Subsystem
  Subsystem1 : Subsystem
  y : Outport  VectorParamsAs1DForOutWhenUnconnected=off
  wires:
  Mux/1 -> y/1
  u/1 -> Demux/1
  Demux/1 -> Subsystem/1(In1)
  Demux/2 -> Subsystem1/1(In1)
  Subsystem/1(Out1) -> Mux/1
  Subsystem1/1(Out1) -> Mux/2

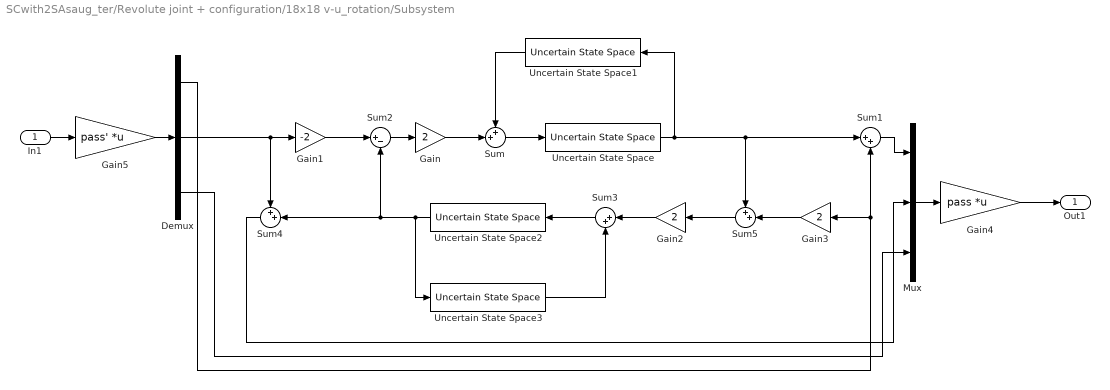
== system SCwith2SAsaug_ter/Revolute joint + configuration/18x18 v-u_rotation/Subsystem ==
  In1 : Inport
  Demux : Demux  Outputs=3
  Gain : Gain  Gain=2
  Gain1 : Gain  Gain=-2
  Gain2 : Gain  Gain=2
  Gain3 : Gain  Gain=2
  Gain4 : Gain  Gain=pass  Multiplication=Matrix(K*u) (u vector)
  Gain5 : Gain  Gain=pass'  Multiplication=Matrix(K*u) (u vector)
  Mux : Mux  Inputs=3
  Sum : Sum  Inputs=++|
  Sum1 : Sum  Inputs=|++
  Sum2 : Sum  Inputs=|+-
  Sum3 : Sum  Inputs=|++
  Sum4 : Sum  Inputs=++|
  Sum5 : Sum  Inputs=++|
  Uncertain State Space{,1..3} (4 alike) : RCTblocks/Uncertain State Space  Tag=USS  USystem=uss(sig4)  UValue=[]  X0=[]  uX0=[]
  Out1 : Outport  VectorParamsAs1DForOutWhenUnconnected=off
  wires:
  Sum5/1 -> Gain2/1
  Sum1/1 -> Mux/1
  Sum2/1 -> Gain/1
  Uncertain State Space1/1 -> Sum/1
  Demux/2 -> Gain1/1, Sum4/1
  Sum/1 -> Uncertain State Space/1
  Gain3/1 -> Sum5/2
  Uncertain State Space/1 -> Sum1/1, Sum5/1, Uncertain State Space1/1
  Gain1/1 -> Sum2/1
  Sum3/1 -> Uncertain State Space2/1
  Sum4/1 -> Mux/2
  Mux/1 -> Gain4/1
  Demux/3 -> Mux/3
  Demux/1 -> Sum1/2, Gain3/1
  Uncertain State Space2/1 -> Sum2/2, Sum4/2, Uncertain State Space3/1
  Gain/1 -> Sum/2
  In1/1 -> Gain5/1
  Gain2/1 -> Sum3/1
  Uncertain State Space3/1 -> Sum3/2
  Gain4/1 -> Out1/1
  Gain5/1 -> Demux/1

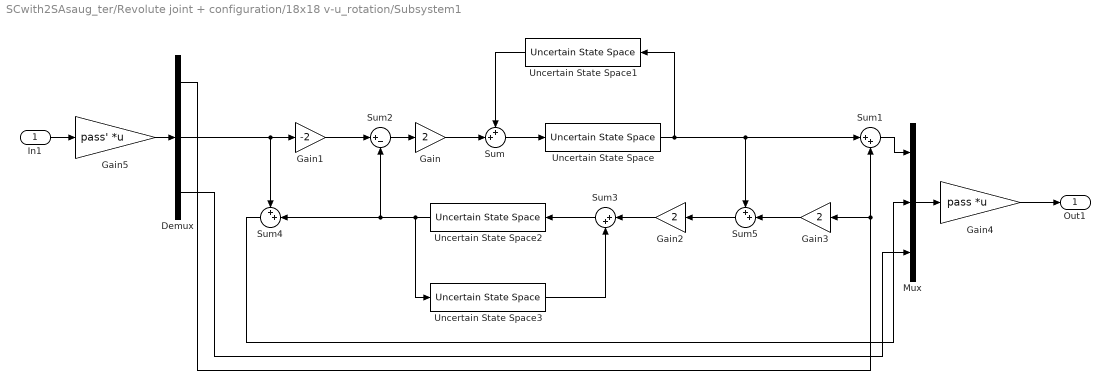
== system SCwith2SAsaug_ter/Revolute joint + configuration/18x18 v-u_rotation/Subsystem1 ==
  In1 : Inport
  Demux : Demux  Outputs=3
  Gain : Gain  Gain=2
  Gain1 : Gain  Gain=-2
  Gain2 : Gain  Gain=2
  Gain3 : Gain  Gain=2
  Gain4 : Gain  Gain=pass  Multiplication=Matrix(K*u) (u vector)
  Gain5 : Gain  Gain=pass'  Multiplication=Matrix(K*u) (u vector)
  Mux : Mux  Inputs=3
  Sum : Sum  Inputs=++|
  Sum1 : Sum  Inputs=|++
  Sum2 : Sum  Inputs=|+-
  Sum3 : Sum  Inputs=|++
  Sum4 : Sum  Inputs=++|
  Sum5 : Sum  Inputs=++|
  Uncertain State Space{,1..3} (4 alike) : RCTblocks/Uncertain State Space  Tag=USS  USystem=uss(sig4)  UValue=[]  X0=[]  uX0=[]
  Out1 : Outport  VectorParamsAs1DForOutWhenUnconnected=off
  wires:
  Gain4/1 -> Out1/1
  Uncertain State Space3/1 -> Sum3/2
  Gain2/1 -> Sum3/1
  In1/1 -> Gain5/1
  Gain/1 -> Sum/2
  Uncertain State Space2/1 -> Uncertain State Space3/1, Sum4/2, Sum2/2
  Demux/1 -> Gain3/1, Sum1/2
  Demux/3 -> Mux/3
  Mux/1 -> Gain4/1
  Sum4/1 -> Mux/2
  Sum3/1 -> Uncertain State Space2/1
  Gain1/1 -> Sum2/1
  Uncertain State Space/1 -> Uncertain State Space1/1, Sum5/1, Sum1/1
  Gain3/1 -> Sum5/2
  Sum/1 -> Uncertain State Space/1
  Demux/2 -> Sum4/1, Gain1/1
  Uncertain State Space1/1 -> Sum/1
  Sum2/1 -> Gain/1
  Sum1/1 -> Mux/1
  Sum5/1 -> Gain2/1
  Gain5/1 -> Demux/1

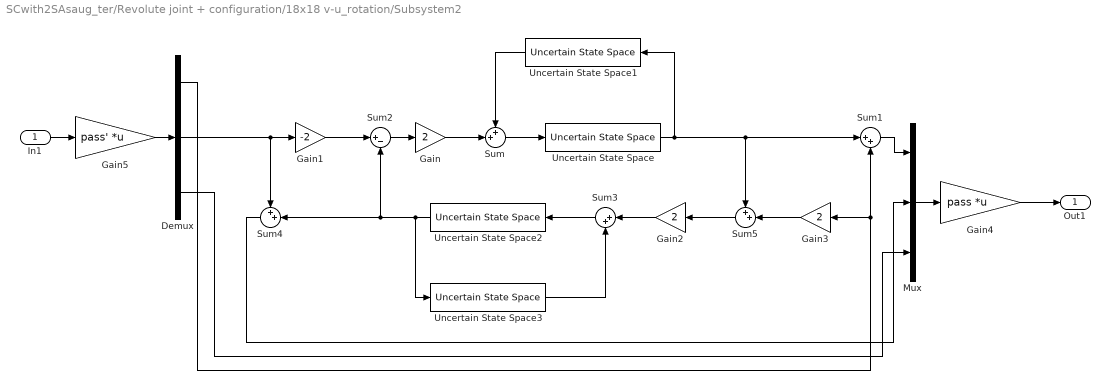
== system SCwith2SAsaug_ter/Revolute joint + configuration/18x18 v-u_rotation/Subsystem2 ==
  In1 : Inport
  Demux : Demux  Outputs=3
  Gain : Gain  Gain=2
  Gain1 : Gain  Gain=-2
  Gain2 : Gain  Gain=2
  Gain3 : Gain  Gain=2
  Gain4 : Gain  Gain=pass  Multiplication=Matrix(K*u) (u vector)
  Gain5 : Gain  Gain=pass'  Multiplication=Matrix(K*u) (u vector)
  Mux : Mux  Inputs=3
  Sum : Sum  Inputs=++|
  Sum1 : Sum  Inputs=|++
  Sum2 : Sum  Inputs=|+-
  Sum3 : Sum  Inputs=|++
  Sum4 : Sum  Inputs=++|
  Sum5 : Sum  Inputs=++|
  Uncertain State Space{,1..3} (4 alike) : RCTblocks/Uncertain State Space  Tag=USS  USystem=uss(sig4)  UValue=[]  X0=[]  uX0=[]
  Out1 : Outport  VectorParamsAs1DForOutWhenUnconnected=off
  wires:
  Gain5/1 -> Demux/1
  Gain4/1 -> Out1/1
  Uncertain State Space3/1 -> Sum3/2
  Gain2/1 -> Sum3/1
  In1/1 -> Gain5/1
  Gain/1 -> Sum/2
  Uncertain State Space2/1 -> Uncertain State Space3/1, Sum4/2, Sum2/2
  Demux/1 -> Gain3/1, Sum1/2
  Demux/3 -> Mux/3
  Mux/1 -> Gain4/1
  Sum4/1 -> Mux/2
  Sum3/1 -> Uncertain State Space2/1
  Gain1/1 -> Sum2/1
  Uncertain State Space/1 -> Uncertain State Space1/1, Sum5/1, Sum1/1
  Gain3/1 -> Sum5/2
  Sum/1 -> Uncertain State Space/1
  Demux/2 -> Sum4/1, Gain1/1
  Uncertain State Space1/1 -> Sum/1
  Sum2/1 -> Gain/1
  Sum1/1 -> Mux/1
  Sum5/1 -> Gain2/1

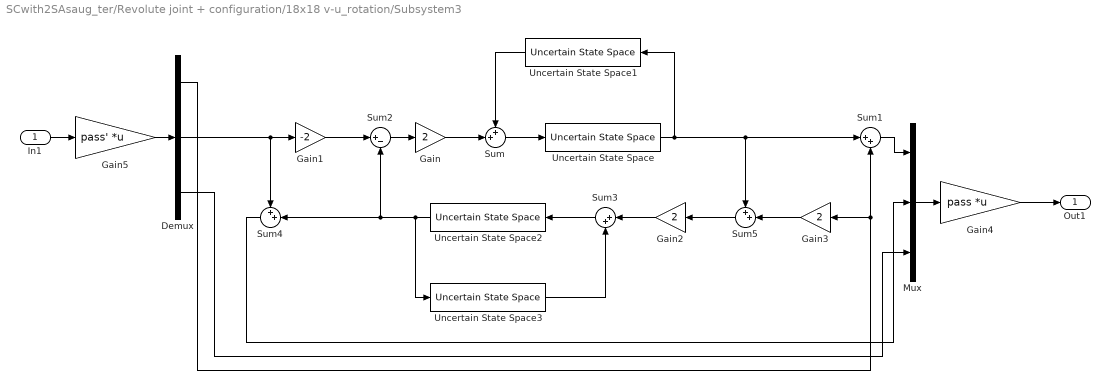
== system SCwith2SAsaug_ter/Revolute joint + configuration/18x18 v-u_rotation/Subsystem3 ==
  In1 : Inport
  Demux : Demux  Outputs=3
  Gain : Gain  Gain=2
  Gain1 : Gain  Gain=-2
  Gain2 : Gain  Gain=2
  Gain3 : Gain  Gain=2
  Gain4 : Gain  Gain=pass  Multiplication=Matrix(K*u) (u vector)
  Gain5 : Gain  Gain=pass'  Multiplication=Matrix(K*u) (u vector)
  Mux : Mux  Inputs=3
  Sum : Sum  Inputs=++|
  Sum1 : Sum  Inputs=|++
  Sum2 : Sum  Inputs=|+-
  Sum3 : Sum  Inputs=|++
  Sum4 : Sum  Inputs=++|
  Sum5 : Sum  Inputs=++|
  Uncertain State Space{,1..3} (4 alike) : RCTblocks/Uncertain State Space  Tag=USS  USystem=uss(sig4)  UValue=[]  X0=[]  uX0=[]
  Out1 : Outport  VectorParamsAs1DForOutWhenUnconnected=off
  wires:
  Gain5/1 -> Demux/1
  Sum5/1 -> Gain2/1
  Sum1/1 -> Mux/1
  Sum2/1 -> Gain/1
  Uncertain State Space1/1 -> Sum/1
  Demux/2 -> Gain1/1, Sum4/1
  Sum/1 -> Uncertain State Space/1
  Gain3/1 -> Sum5/2
  Uncertain State Space/1 -> Sum1/1, Sum5/1, Uncertain State Space1/1
  Gain1/1 -> Sum2/1
  Sum3/1 -> Uncertain State Space2/1
  Sum4/1 -> Mux/2
  Mux/1 -> Gain4/1
  Demux/3 -> Mux/3
  Demux/1 -> Sum1/2, Gain3/1
  Uncertain State Space2/1 -> Sum2/2, Sum4/2, Uncertain State Space3/1
  Gain/1 -> Sum/2
  In1/1 -> Gain5/1
  Gain2/1 -> Sum3/1
  Uncertain State Space3/1 -> Sum3/2
  Gain4/1 -> Out1/1

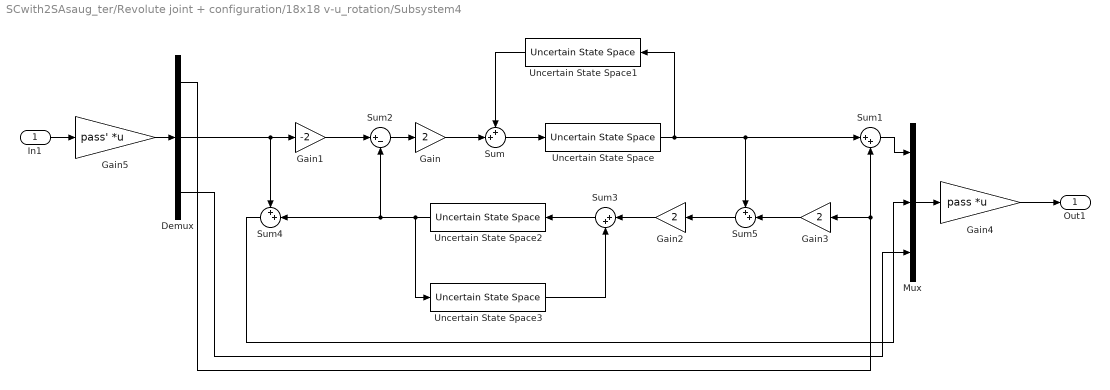
== system SCwith2SAsaug_ter/Revolute joint + configuration/18x18 v-u_rotation/Subsystem4 ==
  In1 : Inport
  Demux : Demux  Outputs=3
  Gain : Gain  Gain=2
  Gain1 : Gain  Gain=-2
  Gain2 : Gain  Gain=2
  Gain3 : Gain  Gain=2
  Gain4 : Gain  Gain=pass  Multiplication=Matrix(K*u) (u vector)
  Gain5 : Gain  Gain=pass'  Multiplication=Matrix(K*u) (u vector)
  Mux : Mux  Inputs=3
  Sum : Sum  Inputs=++|
  Sum1 : Sum  Inputs=|++
  Sum2 : Sum  Inputs=|+-
  Sum3 : Sum  Inputs=|++
  Sum4 : Sum  Inputs=++|
  Sum5 : Sum  Inputs=++|
  Uncertain State Space{,1..3} (4 alike) : RCTblocks/Uncertain State Space  Tag=USS  USystem=uss(sig4)  UValue=[]  X0=[]  uX0=[]
  Out1 : Outport  VectorParamsAs1DForOutWhenUnconnected=off
  wires:
  Sum5/1 -> Gain2/1
  Sum1/1 -> Mux/1
  Sum2/1 -> Gain/1
  Uncertain State Space1/1 -> Sum/1
  Demux/2 -> Gain1/1, Sum4/1
  Sum/1 -> Uncertain State Space/1
  Gain3/1 -> Sum5/2
  Uncertain State Space/1 -> Sum1/1, Sum5/1, Uncertain State Space1/1
  Gain1/1 -> Sum2/1
  Sum3/1 -> Uncertain State Space2/1
  Sum4/1 -> Mux/2
  Mux/1 -> Gain4/1
  Demux/3 -> Mux/3
  Demux/1 -> Sum1/2, Gain3/1
  Uncertain State Space2/1 -> Sum2/2, Sum4/2, Uncertain State Space3/1
  Gain/1 -> Sum/2
  In1/1 -> Gain5/1
  Gain2/1 -> Sum3/1
  Uncertain State Space3/1 -> Sum3/2
  Gain4/1 -> Out1/1
  Gain5/1 -> Demux/1

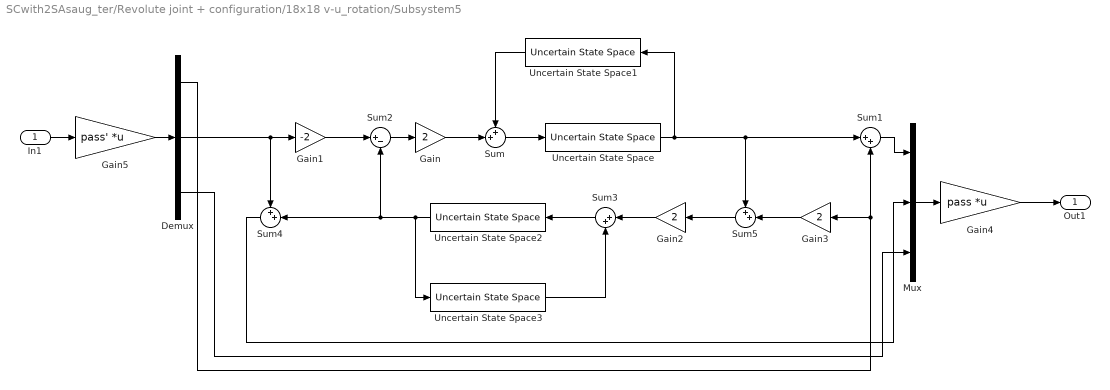
== system SCwith2SAsaug_ter/Revolute joint + configuration/18x18 v-u_rotation/Subsystem5 ==
  In1 : Inport
  Demux : Demux  Outputs=3
  Gain : Gain  Gain=2
  Gain1 : Gain  Gain=-2
  Gain2 : Gain  Gain=2
  Gain3 : Gain  Gain=2
  Gain4 : Gain  Gain=pass  Multiplication=Matrix(K*u) (u vector)
  Gain5 : Gain  Gain=pass'  Multiplication=Matrix(K*u) (u vector)
  Mux : Mux  Inputs=3
  Sum : Sum  Inputs=++|
  Sum1 : Sum  Inputs=|++
  Sum2 : Sum  Inputs=|+-
  Sum3 : Sum  Inputs=|++
  Sum4 : Sum  Inputs=++|
  Sum5 : Sum  Inputs=++|
  Uncertain State Space{,1..3} (4 alike) : RCTblocks/Uncertain State Space  Tag=USS  USystem=uss(sig4)  UValue=[]  X0=[]  uX0=[]
  Out1 : Outport  VectorParamsAs1DForOutWhenUnconnected=off
  wires:
  Gain4/1 -> Out1/1
  Uncertain State Space3/1 -> Sum3/2
  Gain2/1 -> Sum3/1
  In1/1 -> Gain5/1
  Gain/1 -> Sum/2
  Uncertain State Space2/1 -> Uncertain State Space3/1, Sum4/2, Sum2/2
  Demux/1 -> Gain3/1, Sum1/2
  Demux/3 -> Mux/3
  Mux/1 -> Gain4/1
  Sum4/1 -> Mux/2
  Sum3/1 -> Uncertain State Space2/1
  Gain1/1 -> Sum2/1
  Uncertain State Space/1 -> Uncertain State Space1/1, Sum5/1, Sum1/1
  Gain3/1 -> Sum5/2
  Sum/1 -> Uncertain State Space/1
  Demux/2 -> Sum4/1, Gain1/1
  Uncertain State Space1/1 -> Sum/1
  Sum2/1 -> Gain/1
  Sum1/1 -> Mux/1
  Sum5/1 -> Gain2/1
  Gain5/1 -> Demux/1

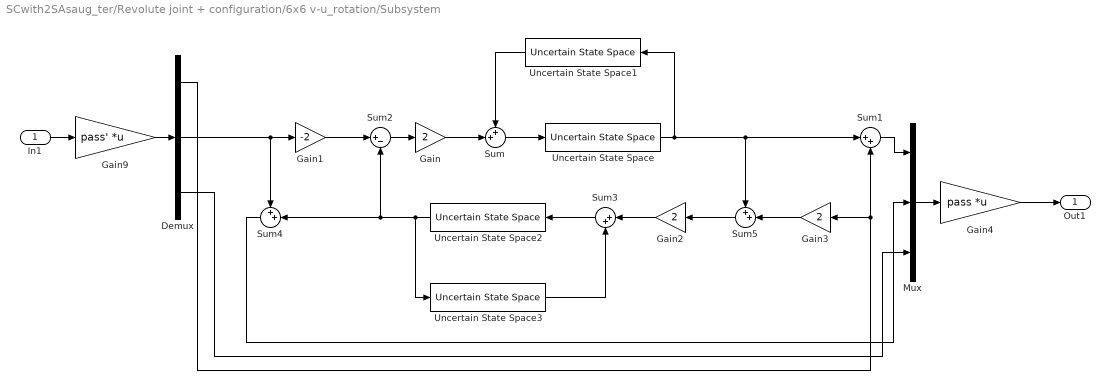
== system SCwith2SAsaug_ter/Revolute joint + configuration/6x6 v-u_rotation/Subsystem ==
  In1 : Inport
  Demux : Demux  Outputs=3
  Gain : Gain  Gain=2
  Gain1 : Gain  Gain=-2
  Gain2 : Gain  Gain=2
  Gain3 : Gain  Gain=2
  Gain4 : Gain  Gain=pass  Multiplication=Matrix(K*u) (u vector)
  Gain9 : Gain  Gain=pass'  Multiplication=Matrix(K*u) (u vector)
  Mux : Mux  Inputs=3
  Sum : Sum  Inputs=++|
  Sum1 : Sum  Inputs=|++
  Sum2 : Sum  Inputs=|+-
  Sum3 : Sum  Inputs=|++
  Sum4 : Sum  Inputs=++|
  Sum5 : Sum  Inputs=++|
  Uncertain State Space{,1..3} (4 alike) : RCTblocks/Uncertain State Space  Tag=USS  USystem=uss(sig4)  UValue=[]  X0=[]  uX0=[]
  Out1 : Outport  VectorParamsAs1DForOutWhenUnconnected=off
  wires:
  Gain4/1 -> Out1/1
  Uncertain State Space3/1 -> Sum3/2
  Gain2/1 -> Sum3/1
  Gain9/1 -> Demux/1
  Gain/1 -> Sum/2
  Uncertain State Space2/1 -> Uncertain State Space3/1, Sum4/2, Sum2/2
  Demux/1 -> Gain3/1, Sum1/2
  Demux/3 -> Mux/3
  Mux/1 -> Gain4/1
  In1/1 -> Gain9/1
  Sum4/1 -> Mux/2
  Sum3/1 -> Uncertain State Space2/1
  Gain1/1 -> Sum2/1
  Uncertain State Space/1 -> Uncertain State Space1/1, Sum5/1, Sum1/1
  Gain3/1 -> Sum5/2
  Sum/1 -> Uncertain State Space/1
  Demux/2 -> Sum4/1, Gain1/1
  Uncertain State Space1/1 -> Sum/1
  Sum2/1 -> Gain/1
  Sum1/1 -> Mux/1
  Sum5/1 -> Gain2/1

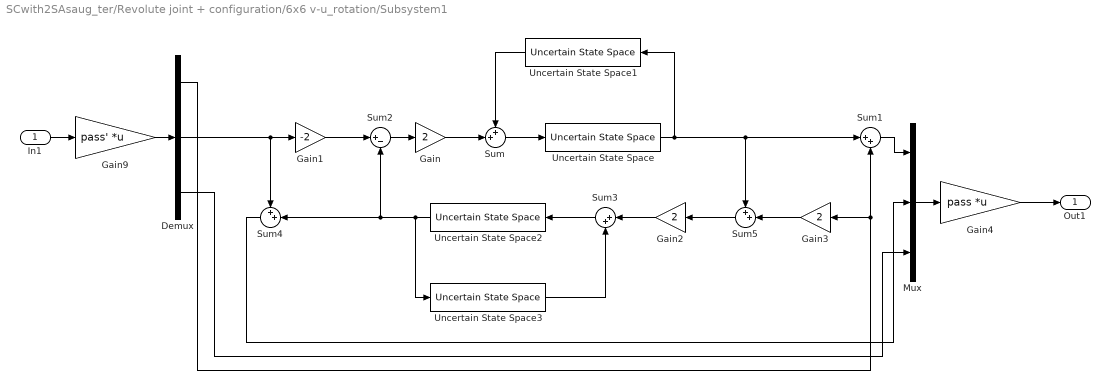
== system SCwith2SAsaug_ter/Revolute joint + configuration/6x6 v-u_rotation/Subsystem1 ==
  In1 : Inport
  Demux : Demux  Outputs=3
  Gain : Gain  Gain=2
  Gain1 : Gain  Gain=-2
  Gain2 : Gain  Gain=2
  Gain3 : Gain  Gain=2
  Gain4 : Gain  Gain=pass  Multiplication=Matrix(K*u) (u vector)
  Gain9 : Gain  Gain=pass'  Multiplication=Matrix(K*u) (u vector)
  Mux : Mux  Inputs=3
  Sum : Sum  Inputs=++|
  Sum1 : Sum  Inputs=|++
  Sum2 : Sum  Inputs=|+-
  Sum3 : Sum  Inputs=|++
  Sum4 : Sum  Inputs=++|
  Sum5 : Sum  Inputs=++|
  Uncertain State Space{,1..3} (4 alike) : RCTblocks/Uncertain State Space  Tag=USS  USystem=uss(sig4)  UValue=[]  X0=[]  uX0=[]
  Out1 : Outport  VectorParamsAs1DForOutWhenUnconnected=off
  wires:
  Sum5/1 -> Gain2/1
  Sum1/1 -> Mux/1
  Sum2/1 -> Gain/1
  Uncertain State Space1/1 -> Sum/1
  Demux/2 -> Gain1/1, Sum4/1
  Sum/1 -> Uncertain State Space/1
  Gain3/1 -> Sum5/2
  Uncertain State Space/1 -> Sum1/1, Sum5/1, Uncertain State Space1/1
  Gain1/1 -> Sum2/1
  Sum3/1 -> Uncertain State Space2/1
  Sum4/1 -> Mux/2
  In1/1 -> Gain9/1
  Mux/1 -> Gain4/1
  Demux/3 -> Mux/3
  Demux/1 -> Sum1/2, Gain3/1
  Uncertain State Space2/1 -> Sum2/2, Sum4/2, Uncertain State Space3/1
  Gain/1 -> Sum/2
  Gain9/1 -> Demux/1
  Gain2/1 -> Sum3/1
  Uncertain State Space3/1 -> Sum3/2
  Gain4/1 -> Out1/1

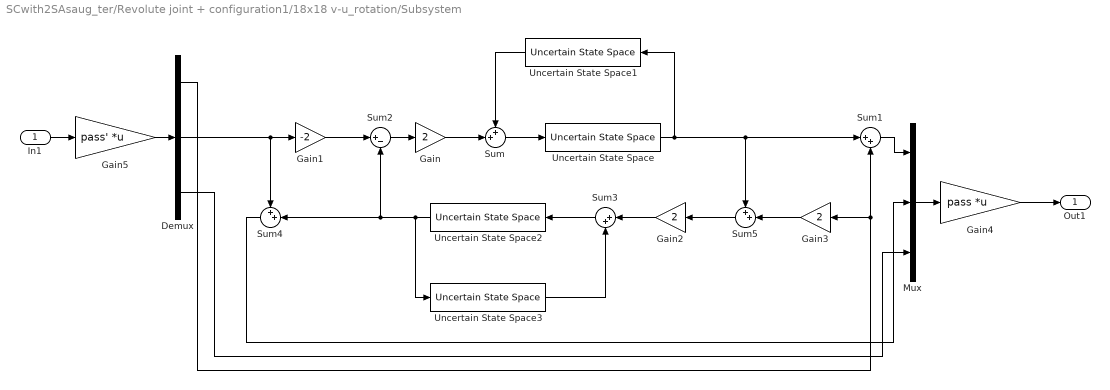
== system SCwith2SAsaug_ter/Revolute joint + configuration1/18x18 v-u_rotation/Subsystem ==
  In1 : Inport
  Demux : Demux  Outputs=3
  Gain : Gain  Gain=2
  Gain1 : Gain  Gain=-2
  Gain2 : Gain  Gain=2
  Gain3 : Gain  Gain=2
  Gain4 : Gain  Gain=pass  Multiplication=Matrix(K*u) (u vector)
  Gain5 : Gain  Gain=pass'  Multiplication=Matrix(K*u) (u vector)
  Mux : Mux  Inputs=3
  Sum : Sum  Inputs=++|
  Sum1 : Sum  Inputs=|++
  Sum2 : Sum  Inputs=|+-
  Sum3 : Sum  Inputs=|++
  Sum4 : Sum  Inputs=++|
  Sum5 : Sum  Inputs=++|
  Uncertain State Space{,1..3} (4 alike) : RCTblocks/Uncertain State Space  Tag=USS  USystem=uss(sig4)  UValue=[]  X0=[]  uX0=[]
  Out1 : Outport  VectorParamsAs1DForOutWhenUnconnected=off
  wires:
  Gain5/1 -> Demux/1
  Gain4/1 -> Out1/1
  Uncertain State Space3/1 -> Sum3/2
  Gain2/1 -> Sum3/1
  In1/1 -> Gain5/1
  Gain/1 -> Sum/2
  Uncertain State Space2/1 -> Uncertain State Space3/1, Sum4/2, Sum2/2
  Demux/1 -> Gain3/1, Sum1/2
  Demux/3 -> Mux/3
  Mux/1 -> Gain4/1
  Sum4/1 -> Mux/2
  Sum3/1 -> Uncertain State Space2/1
  Gain1/1 -> Sum2/1
  Uncertain State Space/1 -> Uncertain State Space1/1, Sum5/1, Sum1/1
  Gain3/1 -> Sum5/2
  Sum/1 -> Uncertain State Space/1
  Demux/2 -> Sum4/1, Gain1/1
  Uncertain State Space1/1 -> Sum/1
  Sum2/1 -> Gain/1
  Sum1/1 -> Mux/1
  Sum5/1 -> Gain2/1

== system SCwith2SAsaug_ter/Revolute joint + configuration1/18x18 v-u_rotation/Subsystem1 ==
  In1 : Inport
  Demux : Demux  Outputs=3
  Gain : Gain  Gain=2
  Gain1 : Gain  Gain=-2
  Gain2 : Gain  Gain=2
  Gain3 : Gain  Gain=2
  Gain4 : Gain  Gain=pass  Multiplication=Matrix(K*u) (u vector)
  Gain5 : Gain  Gain=pass'  Multiplication=Matrix(K*u) (u vector)
  Mux : Mux  Inputs=3
  Sum : Sum  Inputs=++|
  Sum1 : Sum  Inputs=|++
  Sum2 : Sum  Inputs=|+-
  Sum3 : Sum  Inputs=|++
  Sum4 : Sum  Inputs=++|
  Sum5 : Sum  Inputs=++|
  Uncertain State Space{,1..3} (4 alike) : RCTblocks/Uncertain State Space  Tag=USS  USystem=uss(sig4)  UValue=[]  X0=[]  uX0=[]
  Out1 : Outport  VectorParamsAs1DForOutWhenUnconnected=off
  wires:
  Gain5/1 -> Demux/1
  Sum5/1 -> Gain2/1
  Sum1/1 -> Mux/1
  Sum2/1 -> Gain/1
  Uncertain State Space1/1 -> Sum/1
  Demux/2 -> Gain1/1, Sum4/1
  Sum/1 -> Uncertain State Space/1
  Gain3/1 -> Sum5/2
  Uncertain State Space/1 -> Sum1/1, Sum5/1, Uncertain State Space1/1
  Gain1/1 -> Sum2/1
  Sum3/1 -> Uncertain State Space2/1
  Sum4/1 -> Mux/2
  Mux/1 -> Gain4/1
  Demux/3 -> Mux/3
  Demux/1 -> Sum1/2, Gain3/1
  Uncertain State Space2/1 -> Sum2/2, Sum4/2, Uncertain State Space3/1
  Gain/1 -> Sum/2
  In1/1 -> Gain5/1
  Gain2/1 -> Sum3/1
  Uncertain State Space3/1 -> Sum3/2
  Gain4/1 -> Out1/1

== system SCwith2SAsaug_ter/Revolute joint + configuration1/18x18 v-u_rotation/Subsystem2 ==
  In1 : Inport
  Demux : Demux  Outputs=3
  Gain : Gain  Gain=2
  Gain1 : Gain  Gain=-2
  Gain2 : Gain  Gain=2
  Gain3 : Gain  Gain=2
  Gain4 : Gain  Gain=pass  Multiplication=Matrix(K*u) (u vector)
  Gain5 : Gain  Gain=pass'  Multiplication=Matrix(K*u) (u vector)
  Mux : Mux  Inputs=3
  Sum : Sum  Inputs=++|
  Sum1 : Sum  Inputs=|++
  Sum2 : Sum  Inputs=|+-
  Sum3 : Sum  Inputs=|++
  Sum4 : Sum  Inputs=++|
  Sum5 : Sum  Inputs=++|
  Uncertain State Space{,1..3} (4 alike) : RCTblocks/Uncertain State Space  Tag=USS  USystem=uss(sig4)  UValue=[]  X0=[]  uX0=[]
  Out1 : Outport  VectorParamsAs1DForOutWhenUnconnected=off
  wires:
  Sum5/1 -> Gain2/1
  Sum1/1 -> Mux/1
  Sum2/1 -> Gain/1
  Uncertain State Space1/1 -> Sum/1
  Demux/2 -> Gain1/1, Sum4/1
  Sum/1 -> Uncertain State Space/1
  Gain3/1 -> Sum5/2
  Uncertain State Space/1 -> Sum1/1, Sum5/1, Uncertain State Space1/1
  Gain1/1 -> Sum2/1
  Sum3/1 -> Uncertain State Space2/1
  Sum4/1 -> Mux/2
  Mux/1 -> Gain4/1
  Demux/3 -> Mux/3
  Demux/1 -> Sum1/2, Gain3/1
  Uncertain State Space2/1 -> Sum2/2, Sum4/2, Uncertain State Space3/1
  Gain/1 -> Sum/2
  In1/1 -> Gain5/1
  Gain2/1 -> Sum3/1
  Uncertain State Space3/1 -> Sum3/2
  Gain4/1 -> Out1/1
  Gain5/1 -> Demux/1

== system SCwith2SAsaug_ter/Revolute joint + configuration1/18x18 v-u_rotation/Subsystem3 ==
  In1 : Inport
  Demux : Demux  Outputs=3
  Gain : Gain  Gain=2
  Gain1 : Gain  Gain=-2
  Gain2 : Gain  Gain=2
  Gain3 : Gain  Gain=2
  Gain4 : Gain  Gain=pass  Multiplication=Matrix(K*u) (u vector)
  Gain5 : Gain  Gain=pass'  Multiplication=Matrix(K*u) (u vector)
  Mux : Mux  Inputs=3
  Sum : Sum  Inputs=++|
  Sum1 : Sum  Inputs=|++
  Sum2 : Sum  Inputs=|+-
  Sum3 : Sum  Inputs=|++
  Sum4 : Sum  Inputs=++|
  Sum5 : Sum  Inputs=++|
  Uncertain State Space{,1..3} (4 alike) : RCTblocks/Uncertain State Space  Tag=USS  USystem=uss(sig4)  UValue=[]  X0=[]  uX0=[]
  Out1 : Outport  VectorParamsAs1DForOutWhenUnconnected=off
  wires:
  Gain4/1 -> Out1/1
  Uncertain State Space3/1 -> Sum3/2
  Gain2/1 -> Sum3/1
  In1/1 -> Gain5/1
  Gain/1 -> Sum/2
  Uncertain State Space2/1 -> Uncertain State Space3/1, Sum4/2, Sum2/2
  Demux/1 -> Gain3/1, Sum1/2
  Demux/3 -> Mux/3
  Mux/1 -> Gain4/1
  Sum4/1 -> Mux/2
  Sum3/1 -> Uncertain State Space2/1
  Gain1/1 -> Sum2/1
  Uncertain State Space/1 -> Uncertain State Space1/1, Sum5/1, Sum1/1
  Gain3/1 -> Sum5/2
  Sum/1 -> Uncertain State Space/1
  Demux/2 -> Sum4/1, Gain1/1
  Uncertain State Space1/1 -> Sum/1
  Sum2/1 -> Gain/1
  Sum1/1 -> Mux/1
  Sum5/1 -> Gain2/1
  Gain5/1 -> Demux/1
